simulink model "PC_Comm"  (R2024b)
settings: Solver=VariableStepAuto  StartTime=0.0  StopTime=10  RelTol=1e-3
libraries: parrotlib x2, sldrtlib x1
settings Model: Creator=pawel  LastModifiedBy=Pawel

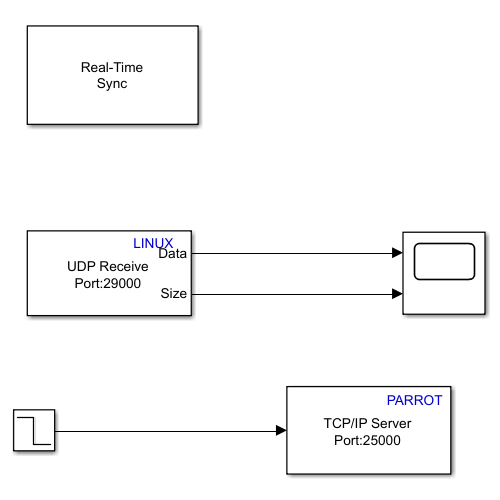
[thumbnail: Simulink's stored preview of the top-level diagram]
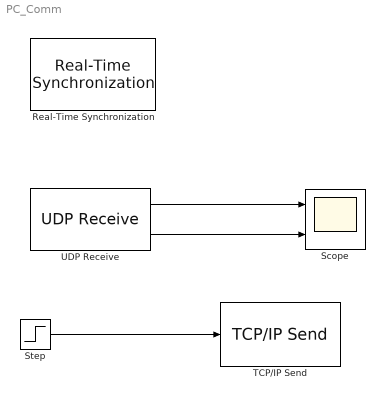
== system PC_Comm ==
  Real-Time Synchronization : sldrtlib/Real-Time Synchronization  SampleTime=0.01  MaxMissedTicks=1000  ShowMissedTicks=off  YieldWhenWaiting=off
  Scope : Scope  NumInputPorts=2
  Step : Step  Time=5  Before=1  After=0  SampleTime=0
  TCP/IP Send : parrotlib/TCP//IP Send  Mode_=Server  LocalServerPort_=25000  RemoteAddr_=192.168.3.2  RemoteServerPort_=25000  SimulateUsing=Code generation  ClientPortBindingSelection_=off  ClientPortToBind_=35000  BlockingMode_=off  BlockTimeout_=0.1
  UDP Receive : parrotlib/UDP Receive  localURL='0.0.0.0'  localPort=29000  remoteURL='0.0.0.0'  remotePort=-1  recvBufferSize=8192  signalDatatype=single  dims=4  isVarSize=off  showBlockingTime=off  blockingTime=0  sampletime=0.005  blockPlatform=LINUX
  wires:
  UDP Receive/1 -> Scope/1
  UDP Receive/2 -> Scope/2
  Step/1 -> TCP/IP Send/1
